simulink model "P413_1_model"  (R2021a)
settings: Solver=VariableStepAuto  StartTime=0.0  StopTime=tspan(end)  RelTol=1e-3
values from neighbouring files (symbols this model uses):
  AR = 10    [P413_1_clima.m]
libraries: HORTISIM x5
settings Model: OrderedModelArguments=off  Creator=djoroya  LastModifiedBy=djoroya

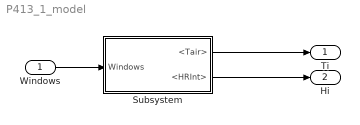
== system P413_1_model ==
  Windows : Inport
  Subsystem : Subsystem
  Ti : Outport
  Hi : Outport  Port=2
  wires:
  Subsystem/1(<Tair>) -> Ti/1
  Subsystem/2(<HRInt>) -> Hi/1
  Windows/1 -> Subsystem/1(Windows)

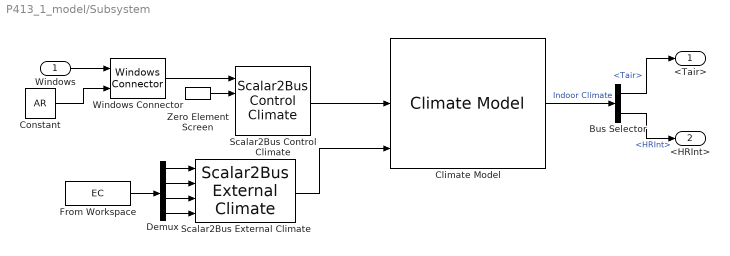
== system P413_1_model/Subsystem ==
  Windows : Inport
  Bus Selector : BusSelector  OutputSignals=Temp.Tair,Gas.HRInt
  Climate Model : HORTISIM/Climate/Models/Climate Model  params=p_ic  x0=x0_ic
      settings: SourceProductName=Horti Simulator
  Constant : Constant  Value=AR
  Demux : Demux
  From Workspace : FromWorkspace  VariableName=EC
  Scalar2Bus External Climate : HORTISIM/Other  Functions/Scalar2Bus External Climate  SystemSampleTime=-1  VariantActivationTime=update diagram  Latency=0  AutoFrameSizeCalculation=off
      settings: SourceProductName=Horti Simulator
  Scalar2Bus Control Climate : HORTISIM/Other  Functions/Scalar2Bus  Control Climate  SystemSampleTime=-1  VariantActivationTime=update diagram  Latency=0  AutoFrameSizeCalculation=off
      settings: SourceProductName=Horti Simulator
  Windows Connector : HORTISIM/Other  Functions/Windows Connector  SystemSampleTime=-1  VariantActivationTime=update diagram  Latency=0  AutoFrameSizeCalculation=off
      settings: SourceProductName=Horti Simulator
  Zero Element Screen : HORTISIM/Other  Functions/Zero Element Screen  SystemSampleTime=-1  VariantActivationTime=update diagram  Latency=0  AutoFrameSizeCalculation=off
      settings: SourceProductName=Horti Simulator
  <Tair> : Outport
  <HRInt> : Outport  Port=2
  wires:
  Bus Selector/2 -> <HRInt>/1  "<HRInt>"
  Windows Connector/1 -> Scalar2Bus Control Climate/1
  Zero Element Screen/1 -> Scalar2Bus Control Climate/2
  From Workspace/1 -> Demux/1
  Demux/4 -> Scalar2Bus External Climate/4
  Demux/1 -> Scalar2Bus External Climate/1
  Bus Selector/1 -> <Tair>/1  "<Tair>"
  Climate Model/1 -> Bus Selector/1  "Indoor Climate"
  Constant/1 -> Windows Connector/2
  Scalar2Bus Control Climate/1 -> Climate Model/2
  Windows/1 -> Windows Connector/1
  Demux/2 -> Scalar2Bus External Climate/2
  Scalar2Bus External Climate/1 -> Climate Model/3
  Demux/3 -> Scalar2Bus External Climate/3
